simulink model "exampleModel"  (R2023b)
settings: Solver=VariableStepAuto  StartTime=0.0  StopTime=1  RelTol=1e-3
libraries: spsThreePhaseVIMeasurementLib x20, spsDistributedParametersLineLib x14, spsThreePhaseSeriesRLCLoadLib x14, spsLoadFlowBusLib x13, spsThreePhaseTransformerTwoWindingsLib x6, spsPower3phPhasorLib x1, spsThreePhaseSourceLib x1, sps_lib x1
settings Model: Creator=shivp  LastModifiedBy=shivp

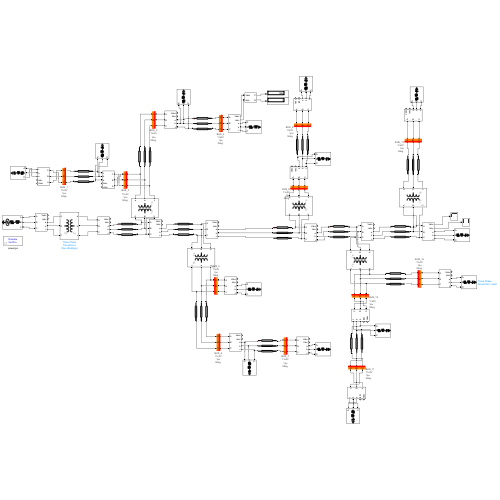
[thumbnail: Simulink's stored preview of the top-level diagram]
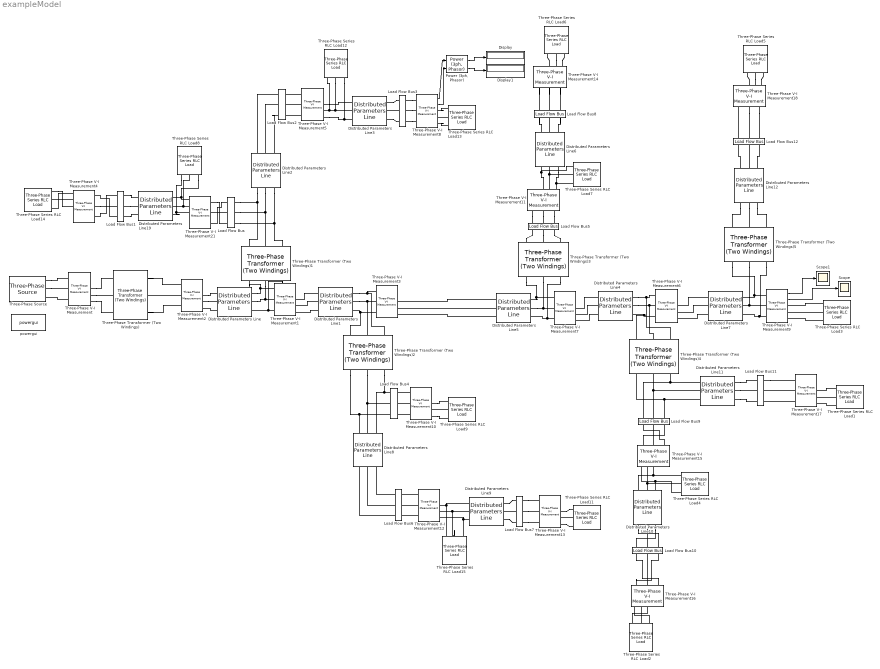
== system exampleModel ==
  Display : Display
  Display1 : Display
  Distributed Parameters Line : spsDistributedParametersLineLib/Distributed Parameters Line  Phases=3  Length=100  Frequency=60  Resistance=[0.01273 0.3864]  Inductance="[0.9337e-3  4.1264e-3]"  Capacitance=[12.74e-9 7.751e-9]  x1=[-0.0006 4.94077504274188 10377.8496125655 -30695.4420255601;-0.00055 5.1486824749925 10859.2496308345 -30528.5274235354;-0.0005 5.3553195468838 11337.9702917476 -30354.0803641771;-0.00045 5.56063527381028 11813.8934781449 -30172.1438896868;-0.0004 5.76457899718851 12286.9017631015 -29982.7628901672;-0.00035 5.96710039695644 12756.878438901 -29785.9840925461;-0.0003 6.16814950398906 13223.7075458309 -29581.8560490475;-0.00025 6.36767671242757 13687.2739007944 -29370.4291252116;-0.0002 6.56563279191888 14147.4631257301 -29151.7554874682;-0.00015 6.76196889976246 14604.1616758324 -28925.8890902654;-0.0001 6.95663659296153 15057.2568675681 -28692.8856627569;-5e-05 7.14958784017568 15506.6369064782 -28452.8026950519]  x2=[-0.0006 200.786537034863 2934.94544321627 -24233.8845899746;-0.00055 216.447490119636 3324.19339842984 -24183.5340234767;-0.0005 232.055038024995 3712.62115866332 -24127.2165318245;-0.00045 247.605329822035 4100.13288517904 -24064.9460105164;-0.0004 263.09452870894 4486.63296525695 -23996.7378238717;-0.00035 278.518812957654 4872.02603578562 -23922.6088012398;-0.0003 293.874376856837 5256.21700679164 -23842.5772328479;-0.00025 309.157431650868 5639.11108490171 -23756.6628652879;-0.0002 324.36420647466 6020.6137967314 -23664.8868966446;-0.00015 339.490949284071 6400.63101219513 -23567.2719712647;-0.0001 354.533927781658 6779.06896773129 -23463.8421741706;-5e-05 369.48943033757 7155.83428943706 -23354.6230251171]  x3=[-0.0006 -6.43137016476401 222.640411310815 145.145208722731;-0.00055 -6.37715378805683 220.308644649267 148.913129004531;-0.0005 -6.32136394407585 217.922520126202 152.644307199984;-0.00045 -6.26401439813027 215.482626482139 156.337822696701;-0.0004 -6.2051193003624 212.989565724328 159.992764175001;-0.00035 -6.14469318225637 210.443952978206 163.608229832763;-0.0003 -6.08275095305263 207.846416335627 167.183327607937;-0.00025 -6.01930789606939 205.19759669989 170.717175398642;-0.0002 -5.95437966493162 202.498147627605 174.208901280813;-0.00015 -5.88798227970884 199.748735167437 177.657643723337;-0.0001 -5.8201321229623 196.950037695771 181.06255180062;-5e-05 -5.75084593570292 194.102745749331 184.422785402543]  x4=[-0.0006 6.58204531239141 -184.73619828775 -350.009915302539;-0.00055 6.54912957666029 -179.156548049083 -353.150209345104;-0.0005 6.51459794120286 -173.532693612961 -356.203368857813;-0.00045 6.47845892618346 -167.866022581315 -359.168640519242;-0.0004 6.44072144836329 -162.157933120431 -362.045292692978;-0.00035 6.40139481890031 -156.409833615971 -364.832615608143;-0.0003 6.3604887410519 -150.623142325477 -367.529921534514;-0.00025 6.31801330778067 -144.799287028436 -370.136544952214;-0.0002 6.2739789992642 -138.939704673999 -372.651842715919;-0.00015 6.22839668030924 -133.045841026433 -375.075194213544;-0.0001 6.1812775976709 -127.119150308402 -377.406001519367;-5e-05 6.13263337727778 -121.161094842157 -379.643689541562]  x5=0.000565541566995742  V1=[14.16 3.243e+04 3.24e+04;314.2 314.2 314.2;0.3671 0.4058 -1.164]  V2=[1019 2.498e+04 2.442e+04;314.2 314.2 314.2;0.2092 0.1979 -1.367]  I1=[7.275 266.6 281.4;314.2 314.2 314.2;-1.074 2.234 0.6222]  I2=[6.892 399.1 404.5;314.2 314.2 314.2;1.883 -0.4011 -2.016]  nHarmo=1  Measurements=None  Decoupling=off  VsMag0=0  VrMag0=0  VsAngle0=0  VrAngle0=0  IsMag0=0  IrMag0=0  IsAngle0=0  IrAngle0=0
      settings: LibrarySourceBlock=sps_lib/Power Grid Elements/Distributed Parameters Line
  Distributed Parameters Line1 : spsDistributedParametersLineLib/Distributed Parameters Line  Phases=3  Length=100  Frequency=60  Resistance=[0.01273 0.3864]  Inductance="[0.9337e-3  4.1264e-3]"  Capacitance=[12.74e-9 7.751e-9]  x1=[-0.0006 200.786537034863 2934.94544321627 -24233.8845899746;-0.00055 216.447490119636 3324.19339842984 -24183.5340234767;-0.0005 232.055038024995 3712.62115866332 -24127.2165318245;-0.00045 247.605329822035 4100.13288517904 -24064.9460105164;-0.0004 263.09452870894 4486.63296525695 -23996.7378238717;-0.00035 278.518812957654 4872.02603578562 -23922.6088012398;-0.0003 293.874376856837 5256.21700679164 -23842.5772328479;-0.00025 309.157431650868 5639.11108490171 -23756.6628652879;-0.0002 324.36420647466 6020.6137967314 -23664.8868966446;-0.00015 339.490949284071 6400.63101219513 -23567.2719712647;-0.0001 354.533927781658 6779.06896773129 -23463.8421741706;-5e-05 369.48943033757 7155.83428943706 -23354.6230251171]  x2=[-0.0006 -9.4511266483093 -2063.31583954316 -18449.4745269581;-0.00055 0.255298879042691 -1766.85331668026 -18477.1445161307;-0.0005 9.96166141521642 -1469.95484919947 -18500.2555463735;-0.00045 19.6655660604955 -1172.69369235505 -18518.8019153854;-0.0004 29.3646185216113 -875.143190889432 -18532.7790471275;-0.00035 39.0564257024991 -577.376760936508 -18542.1834929517;-0.0003 48.7385962947587 -279.467871907298 -18547.0129324516;-0.00025 58.4087413676738 18.5099716375379 -18547.2661740353;-0.0002 68.0644749576452 316.483248123843 -18542.9431552193;-0.00015 77.7034146568914 614.378437104314 -18534.0449426437;-0.0001 87.3231822012721 912.122037398571 -18520.5737318095;-5e-05 96.9214040570896 1209.64058522847 -18502.5328465362]  x3=[-0.0006 2.35637752335621 200.746585968119 86.1206764107603;-0.00055 2.34192006818089 199.357183928959 89.1848960264509;-0.0005 2.32688477927164 197.918593487711 92.2271106035492;-0.00045 2.31127536636103 196.431169595039 95.2465695211299;-0.0004 2.29509568083813 194.895279250532 98.2425277728863;-0.00035 2.27834971479823 193.311301412151 101.214246150949;-0.0003 2.26104160005789 191.679626902725 104.160991428276;-0.00025 2.24317560713542 190.000658313525 107.082036539562;-0.0002 2.22475614419726 188.274809904927 109.976660760634;-0.00015 2.20578775597025 186.502507504201 112.84414988628;-0.0001 2.18627512262036 184.684188400446 115.683796406465;-5e-05 2.16622305859791 182.820301236692 118.494899680901]  x4=[-0.0006 -2.29653629180572 -206.26394733368 -243.453316618494;-0.00055 -2.2482852490429 -202.346734894282 -246.568009410702;-0.0005 -2.19947947553669 -198.379596425829 -249.621865236064;-0.00045 -2.15013101338141 -194.363510760375 -252.61413060135;-0.0004 -2.10025203857168 -190.299468806964 -255.544067209858;-0.00035 -2.04985485799818 -186.188473307137 -258.410952143569;-0.0003 -1.9989519064111 -182.03153858752 -261.214078041525;-0.00025 -1.94755574335208 -177.829690309553 -263.952753274354;-0.0002 -1.89567905005529 -173.583965216424 -266.626302114923;-0.00015 -1.84333462631855 -169.295410877271 -269.23406490506;-0.0001 -1.79053538734517 -164.965085428706 -271.775398218317;-5e-05 -1.73729436055733 -160.594057313737 -274.249675018726]  x5=0.000565541566995742  V1=[1019 2.498e+04 2.442e+04;314.2 314.2 314.2;0.2092 0.1979 -1.367]  V2=[618 1.897e+04 1.855e+04;314.2 314.2 314.2;-0.004469 -0.02884 -1.594]  I1=[2.523 218.7 213.9;314.2 314.2 314.2;1.947 2.059 0.4946]  I2=[3.821 322.4 315.2;314.2 314.2 314.2;-0.634 -0.6141 -2.179]  nHarmo=1  Measurements=None  Decoupling=off  VsMag0=0  VrMag0=0  VsAngle0=0  VrAngle0=0  IsMag0=0  IrMag0=0  IsAngle0=0  IrAngle0=0
      settings: LibrarySourceBlock=sps_lib/Power Grid Elements/Distributed Parameters Line
  Distributed Parameters Line10 : spsDistributedParametersLineLib/Distributed Parameters Line  Phases=3  Length=100  Frequency=60  Resistance=[0.01273 0.3864]  Inductance="[0.9337e-3  4.1264e-3]"  Capacitance=[12.74e-9 7.751e-9]  x1=[-0.0006 -31.2534203294304 -3259.14632862606 -2098.05285456964;-0.00055 -31.121311210234 -3225.34530243776 -2147.64844888902;-0.0005 -30.9815233731746 -3190.74847055797 -2196.71414308959;-0.00045 -30.8340913088094 -3155.36436923726 -2245.23783094549;-0.0004 -30.6790513937942 -3119.20172897317 -2293.20753996283;-0.00035 -30.5164418819081 -3082.26947235608 -2340.61143433367;-0.0003 -30.3463028946149 -3044.57671186767 -2387.43781785642;-0.00025 -30.1686764111639 -3006.13274763258 -2433.67513682161;-0.0002 -29.9836062582321 -2966.94706512375 -2479.31198286265;-0.00015 -29.7911380991104 -2927.02933282198 -2524.33709577066;-0.0001 -29.5913194224371 -2886.38939983042 -2568.73936627276;-5e-05 -29.3841995304807 -2845.03729344442 -2612.5078387731]  x2=[-0.0006 -31.9626959429525 -2654.70923607677 -3040.23236273384;-0.00055 -31.1478015841112 -2605.78900431863 -3080.34012920064;-0.0005 -30.3252219713036 -2556.22583311494 -3119.68786783269;-0.00045 -29.4951600637406 -2506.03195143655 -3158.26587016424;-0.0004 -28.6578206667774 -2455.2197438727 -3196.06461765047;-0.00035 -27.8134103813809 -2403.8017475753 -3233.07478401604;-0.0003 -26.9621375531538 -2351.79064916554 -3269.28723755619;-0.00025 -26.1042122209286 -2299.19928160369 -3304.69304338987;-0.0002 -25.2398460649435 -2246.04062102277 -3339.28346566427;-0.00015 -24.3692523546139 -2192.32778352684 -3373.0499697103;-0.0001 -23.4926458959107 -2138.07402195483 -3405.98422414832;-5e-05 -22.6102429783607 -2083.29272261059 -3438.07810294388]  x3=[-0.0006 -0.345240872027474 -44.4331799500981 -28.7697264815166;-0.00055 -0.343762803006474 -43.96968801251 -29.4458458734078;-0.0005 -0.342199915657665 -43.4953472123374 -30.1146999434374;-0.00045 -0.340552595600116 -43.010274586075 -30.7761236618718;-0.0004 -0.338821249285399 -42.5145898181351 -31.4299538323058;-0.00035 -0.337006303897313 -42.008415211317 -32.076029131928;-0.0003 -0.335108207246473 -41.4918756566308 -32.714190151326;-0.00025 -0.333127427659828 -40.9650986024827 -33.344279433817;-0.0002 -0.331064453865099 -40.4282140232284 -33.9661415142989;-0.00015 -0.328919794870204 -39.8813543871042 -34.5796229576084;-0.0001 -0.326693979837657 -39.3246546235424 -35.1845723963791;-5e-05 -0.324387557954011 -38.7582520898798 -35.7808405683891]  x4=[-0.0006 0.254867368595789 21.6219762320696 11.0058318246452;-0.00055 0.254519474301124 21.4445338180896 11.3354955184404;-0.0005 0.254108781134632 21.2618002862713 11.662362348333;-0.00045 0.253635390428706 21.0738207233796 11.9863516648239;-0.0004 0.25309941898542 20.8806415105588 12.307383528397;-0.00035 0.252500999047707 20.6823103118889 12.6253787292439;-0.0003 0.251840278266732 20.4788760626257 12.940258806807;-0.00025 0.251117419665462 20.270388957126 13.2519460691387;-0.0002 0.250332601598441 20.0569004364634 13.5603636120709;-0.00015 0.249486017707782 19.8384631757361 13.86543533819;-0.0001 0.248577876875393 19.6151310710694 14.1670859756123;-5e-05 0.247608403171435 19.3869592263184 14.4652410965568]  x5=0.000565541566995742  V1=[32.3 3891 3805;314.2 314.2 314.2;-1.304 -0.9126 -2.477]  V2=[60.72 4077 3986;314.2 314.2 314.2;-0.5435 -0.629 -2.194]  I1=[0.3571 53.15 51.96;314.2 314.2 314.2;-1.301 -0.9099 -2.475]  I2=[0.2557 24.32 23.78;314.2 314.2 314.2;1.661 2.126 0.5614]  nHarmo=1  Measurements=None  Decoupling=off  VsMag0=0  VrMag0=0  VsAngle0=0  VrAngle0=0  IsMag0=0  IrMag0=0  IsAngle0=0  IrAngle0=0
      settings: LibrarySourceBlock=sps_lib/Power Grid Elements/Distributed Parameters Line
  Distributed Parameters Line11 : spsDistributedParametersLineLib/Distributed Parameters Line  Phases=3  Length=100  Frequency=60  Resistance=[0.01273 0.3864]  Inductance="[0.9337e-3  4.1264e-3]"  Capacitance=[12.74e-9 7.751e-9]  x1=[-0.0006 -31.253420329437 187.39390622673 3871.52994252577;-0.00055 -31.1213112102406 247.245463917248 3867.05519233241;-0.0005 -30.9815233731812 307.036017489159 3861.62630413434;-0.00045 -30.834091308816 366.750814518032 3855.24461742848;-0.0004 -30.6790513938007 426.375121271234 3847.91170680052;-0.00035 -30.5164418819145 485.89422634325 3839.62938153646;-0.0003 -30.3463028946213 545.293444285507 3830.39968517611;-0.00025 -30.1686764111703 604.558119229787 3820.22489500894;-0.0002 -29.9836062582384 663.673628504345 3809.10752151218;-0.00015 -29.7911380991167 722.625386241831 3797.05030773138;-0.0001 -29.5913194224434 781.398846978137 3784.05622860364;-5e-05 -29.384199530487 839.979509241274 3770.12849022354]  x2=[-0.0006 -31.9626959429525 1305.5638414967 3819.16181947058;-0.00055 -31.1478015841112 1364.75830202508 3796.84953924242;-0.0005 -30.3252219713036 1423.61602886375 3773.60044320392;-0.00045 -29.4951600637406 1482.12249974932 3749.42026772166;-0.0004 -28.6578206667774 1540.26327908556 3724.31497889212;-0.00035 -27.8134103813809 1598.02402150513 3698.29077106966;-0.0003 -26.9621375531538 1655.39047540914 3671.35406533815;-0.00025 -26.1042122209286 1712.34848648349 3643.51150792666;-0.0002 -25.2398460649435 1768.88400119122 3614.76996856963;-0.00015 -24.3692523546139 1824.98307024003 3585.13653881182;-0.0001 -23.4926458959107 1880.63185202407 3554.61853025861;-5e-05 -22.6102429783607 1935.81661603912 3523.22347277195]  x3=[-0.0006 -0.345240872027459 2.69872401787422 52.8651258484685;-0.00055 -0.343762803006458 3.51600655603732 52.8017897520135;-0.0005 -0.342199915657649 4.33242157219386 52.7254256040274;-0.00045 -0.340552595600099 5.14776762815486 52.636052246221;-0.0004 -0.338821249285382 5.96184354948133 52.5336917301329;-0.00035 -0.337006303897295 6.77444847512094 52.418369311689;-0.0003 -0.335108207246455 7.58538190696757 52.2901134449703;-0.00025 -0.333127427659809 8.39444375933115 52.1489557751928;-0.0002 -0.33106445386508 9.20143440830588 51.9949311308993;-0.00015 -0.328919794870184 10.0061547410244 51.8280775153662;-0.0001 -0.326693979837637 10.8084062047858 51.6484360972263;-5e-05 -0.324387557953991 11.6079908560459 51.4560512003116]  x4=[-0.0006 0.254867368595761 1.27965816611283 -24.228096609318;-0.00055 0.254519474301095 0.905439825590797 -24.2392588180001;-0.0005 0.254108781134602 0.530998081340184 -24.2444403522685;-0.00045 0.253635390428675 0.156425321258497 -24.2436399336574;-0.0004 0.253099418985388 -0.21818603443057 -24.2368577596581;-0.00035 0.252500999047674 -0.592743555980428 -24.2240955036704;-0.0003 0.251840278266699 -0.967154826927261 -24.2053563145901;-0.00025 0.251117419665428 -1.3413274668924 -24.1806448160318;-0.0002 0.250332601598405 -1.71516915437579 -24.1499671051878;-0.00015 0.249486017707745 -2.08858764953497 -24.1133307513243;-0.0001 0.248577876875355 -2.46149081694384 -24.0707447939135;-5e-05 0.247608403171397 -2.8337866483257 -24.022219740403]  x5=0.000565541566995742  V1=[32.3 3817 3880;314.2 314.2 314.2;-1.304 0.1293 1.717]  V2=[60.72 3998 4064;314.2 314.2 314.2;-0.5435 0.4128 2]  I1=[0.3571 52.12 52.99;314.2 314.2 314.2;-1.301 0.1319 1.719]  I2=[0.2557 23.85 24.24;314.2 314.2 314.2;1.661 -3.115 -1.528]  nHarmo=1  Measurements=None  Decoupling=off  VsMag0=0  VrMag0=0  VsAngle0=0  VrAngle0=0  IsMag0=0  IrMag0=0  IsAngle0=0  IrAngle0=0
      settings: LibrarySourceBlock=sps_lib/Power Grid Elements/Distributed Parameters Line
  Distributed Parameters Line12 : spsDistributedParametersLineLib/Distributed Parameters Line  Phases=3  Length=100  Frequency=60  Resistance=[0.01273 0.3864]  Inductance="[0.9337e-3  4.1264e-3]"  Capacitance=[12.74e-9 7.751e-9]  x1=[-0.0006 -13.9948706374657 -919.303427512541 3469.68312771773;-0.00055 -14.107672519494 -865.812114028127 3483.03655716339;-0.0005 -14.2169935444258 -812.107174360002 3495.53059945637;-0.00045 -14.3228067389339 -758.201859398424 3507.16217187868;-0.0004 -14.4250859951959 -704.109469473257 3517.92840451387;-0.00035 -14.5238060773359 -649.843351072314 3527.82664095514;-0.0003 -14.6189426276506 -595.416893548309 3536.85443896076;-0.00025 -14.7104721726198 -540.843525815234 3545.00957105666;-0.0002 -14.798372128698 -486.136713034981 3552.29002508601;-0.00015 -14.8826208078863 -431.309953295005 3558.69400470573;-0.0001 -14.9631974230836 -376.376774277884 3564.21992982967;-5e-05 -15.0400820932159 -321.350729923556 3568.86643701849]  x2=[-0.0006 -28.5037047462179 71.306703847752 3746.70935246665;-0.00055 -28.3711521317178 129.213636434848 3744.1363373644;-0.0005 -28.2315993599558 187.088687490618 3740.63951264562;-0.00045 -28.0850808634902 244.917577212219 3736.21974109948;-0.0004 -27.9316327935677 302.686037186423 3730.87811323849;-0.00035 -27.7712930112033 360.379813910139 3724.61594702938;-0.0003 -27.6041010778393 417.984672307252 3717.43478756796;-0.00025 -27.4300982455832 475.486399240912 3709.33640669789;-0.0002 -27.2493274470305 532.870807020415 3700.32280257345;-0.00015 -27.0618332846706 590.123736901803 3690.3961991666;-0.0001 -26.8676620198827 647.231062581322 3679.55904571818;-5e-05 -26.6668615615208 704.178693680874 3667.81401613366]  x3=[-0.0006 -0.154985241892026 -12.4308431243015 47.4184090726545;-0.00055 -0.156224478566297 -11.6997862553303 47.5987825840961;-0.0005 -0.157425169188118 -10.9658426391682 47.767411808171;-0.00045 -0.158587017505046 -10.2291933654204 47.9242551381413;-0.0004 -0.159709736848393 -9.49002019127238 48.0692738752623;-0.00035 -0.160793050203961 -8.74850549664436 48.2024322383305;-0.0003 -0.161836690280388 -8.00483223919175 48.3236973725125;-0.00025 -0.162840399575104 -7.25918390916299 48.4330393574507;-0.0002 -0.163803930437857 -6.51174448412615 48.5304312146467;-0.00015 -0.164727045131826 -5.76269838357518 48.6158489141168;-0.0001 -0.165609515892272 -5.01223042342716 48.689271380322;-5e-05 -0.166451124982741 -4.26052577042177 48.7506804973673]  x4=[-0.0006 0.098898525106131 7.89349892269427 -21.004432828506;-0.00055 0.100084430701719 7.56999516148253 -21.1224544565239;-0.0005 0.101245641961626 7.24462361723696 -21.2352644349667;-0.00045 0.102381872374351 6.91746457051747 -21.3428349296603;-0.0004 0.10349284159204 6.58859874292344 -21.4451393991946;-0.00035 0.104578275499663 6.25810727717692 -21.5421526014727;-0.0003 0.105637906282645 5.92607171710183 -21.6338505999386;-0.00025 0.106671472492945 5.59257398750425 -21.7202107694831;-0.0002 0.107678719113567 5.25769637395874 -21.8012118020268;-0.00015 0.10865939762148 4.92152150250556 -21.8768337117769;-0.0001 0.109613266048934 4.58413231926394 -21.9470578401587;-5e-05 0.11054008904317 4.24561206996638 -22.0118668604193]  x5=0.000565541566995742  V1=[15.78 3520 3579;314.2 314.2 314.2;-2.04 -0.1841 1.403]  V2=[29.66 3688 3749;314.2 314.2 314.2;-1.279 0.09948 1.687]  I1=[0.1745 48.08 48.88;314.2 314.2 314.2;-2.037 -0.1814 1.406]  I2=[0.1249 22 22.36;314.2 314.2 314.2;0.9246 2.855 -1.841]  nHarmo=1  Measurements=None  Decoupling=off  VsMag0=0  VrMag0=0  VsAngle0=0  VrAngle0=0  IsMag0=0  IrMag0=0  IsAngle0=0  IrAngle0=0
      settings: LibrarySourceBlock=sps_lib/Power Grid Elements/Distributed Parameters Line
  Distributed Parameters Line19 : spsDistributedParametersLineLib/Distributed Parameters Line  Phases=3  Length=100  Frequency=60  Resistance=[0.01273 0.3864]  Inductance="[0.9337e-3  4.1264e-3]"  Capacitance=[12.74e-9 7.751e-9]  x1=[-0.0006 -96.5409517097259 5973.89106489545 4979.15177398064;-0.00055 -94.1120389876083 6051.66956004539 4881.77212845539;-0.0005 -91.6599055280992 6127.95489628446 4783.18797870496;-0.00045 -89.1851563584376 6202.72825134744 4683.42364889317;-0.0004 -86.6884020859507 6275.97117602781 4582.50375437559;-0.00035 -84.1702587473955 6347.66559872986 4480.45319562609;-0.0003 -81.631347656961 6417.79382992759 4377.29715209302;-0.00025 -79.0722952529682 6486.3385665293 4273.06107598659;-0.0002 -76.4937329433059 6553.28289614688 4167.77068599884;-0.00015 -73.8962969496402 6618.61030126871 4061.45196095801;-0.0001 -71.2806281504361 6682.3046633351 3954.13113341862;-5e-05 -68.6473719228309 6744.35026671528 3845.834683189]  x2=[-0.0006 68.0412810259189 7473.03807820244 3202.33927910117;-0.00055 73.2889661597856 7523.58354001883 3081.70422208403;-0.0005 78.5185683378987 7572.27267017452 2960.30880066263;-0.00045 83.728797234173 7619.0934553552 2838.18296734071;-0.0004 88.9183673025907 7664.0343432327 2715.35685484025;-0.00035 94.0859980943905 7707.08424531542 2591.86076866661;-0.0003 99.2304145739996 7748.23253968419 2467.72517963114;-0.00025 104.350347433629 7787.46907361308 2342.98071633297;-0.0002 109.444533406457 7824.78416607446 2217.65815760182;-0.00015 114.511715578321 7860.16861012761 2091.78842490381;-0.0001 119.550643697841 7893.61367519045 1965.40257471205;-5e-05 124.560074484904 7925.11110919361 1838.53179084394]  x3=[-0.0006 -1.06184548840488 81.7697475785311 67.7761452130824;-0.00055 -1.0349383777841 82.8285325706211 66.44337440146;-0.0005 -1.00777591160473 83.8668808616892 65.0942096814175;-0.00045 -0.980364791798835 84.8845362548318 63.7289839391618;-0.0004 -0.952711781650081 85.8812476588081 62.3480340237163;-0.00035 -0.924823704124937 86.8567691499932 60.9517006638091;-0.0003 -0.896707440189235 87.8108600330563 59.540328383803;-0.00025 -0.868369927110387 88.7432849003484 58.1142654186893;-0.0002 -0.839818156745723 89.6538136899856 56.6738636281659;-0.00015 -0.81105917381735 90.5422217426136 55.2194784098215;-0.0001 -0.782100074173978 91.408289856839 53.7514686114462;-5e-05 -0.752948003040117 92.2518043433138 52.2701964424916]  x4=[-0.0006 0.96623222764616 -33.9273887860384 -34.9003273923412;-0.00055 0.949390278302067 -34.4714181256832 -34.3446948123242;-0.0005 0.932314081112835 -35.0069421587123 -33.7805881927728;-0.00045 0.915007849374603 -35.5338287525838 -33.2081467185547;-0.0004 0.897475853141095 -36.0519479059148 -32.627511631038;-0.00035 0.879722418170043 -36.5611717805569 -32.0388261932422;-0.0003 0.861751924855877 -37.0613747331386 -31.4422356544905;-0.00025 0.843568807148924 -37.5524333460662 -30.8378872145714;-0.0002 0.825177551461397 -38.0342264579748 -30.2259299874192;-0.00015 0.806582695560445 -38.5066351936232 -29.606514964323;-0.0001 0.787788827448518 -38.9695429932248 -28.979794976671;-5e-05 0.768800584231356 -39.4228356412065 -28.3459246582426]  x5=0.000565541566995742  V1=[181.7 7789 7921;314.2 314.2 314.2;-0.5495 0.9542 2.542]  V2=[341.5 8160 8298;314.2 314.2 314.2;0.2114 1.238 2.826]  I1=[2.008 106.4 108.2;314.2 314.2 314.2;-0.5463 0.9569 2.545]  I2=[1.438 48.67 49.5;314.2 314.2 314.2;2.415 -2.29 -0.7024]  nHarmo=1  Measurements=None  Decoupling=off  VsMag0=0  VrMag0=0  VsAngle0=0  VrAngle0=0  IsMag0=0  IrMag0=0  IsAngle0=0  IrAngle0=0
      settings: LibrarySourceBlock=sps_lib/Power Grid Elements/Distributed Parameters Line
  Distributed Parameters Line2 : spsDistributedParametersLineLib/Distributed Parameters Line  Phases=3  Length=100  Frequency=60  Resistance=[0.01273 0.3864]  Inductance="[0.9337e-3  4.1264e-3]"  Capacitance=[12.74e-9 7.751e-9]  x1=[-0.0006 68.0412810259189 963.211871862868 -8073.01045872234;-0.00055 73.2889661597856 1092.95762673489 -8056.46658419278;-0.0005 78.5185683378987 1222.43371066678 -8037.93489708508;-0.00045 83.728797234173 1351.60817737224 -8017.41996981571;-0.0004 88.9183673025907 1480.44915498448 -7994.92686413603;-0.00035 94.0859980943905 1608.92485392017 -7970.46112988328;-0.0003 99.2304145739996 1737.00357472301 -7944.0288036113;-0.00025 104.350347433629 1864.65371588512 -7915.63640710108;-0.0002 109.444533406457 1991.84378164426 -7885.29094575162;-0.00015 114.511715578321 2118.54238975487 -7852.99990685144;-0.0001 119.550643697841 2244.71827923124 -7818.7712577312;-5e-05 124.560074484904 2370.34031806066 -7782.61344379791]  x2=[-0.0006 2087.33596012298 -628.82209039192 -6402.97812602283;-0.00055 2162.21893486438 -491.528832065564 -6413.85133834206;-0.0005 2236.56841443757 -354.114296354799 -6423.14202881608;-0.00045 2310.366054221 -216.612388240135 -6430.84790510602;-0.0004 2383.59364575129 -79.0570342599129 -6436.96706590223;-0.00035 2456.23312121598 58.5178258605571 -6441.49800139332;-0.0003 2528.2665579114 196.078247583117 -6444.43959363878;-0.00025 2599.67618266493 333.590289932067 -6445.79111684472;-0.0002 2670.44437622018 471.020023868596 -6445.55223754303;-0.00015 2740.55367758431 608.333540662258 -6443.72301467359;-0.0001 2809.98678833628 745.496960257453 -6440.30389956978;-5e-05 2878.72657689496 882.476439632814 -6435.29573584708]  x3=[-0.0006 -26.6808406064646 -16.3698197682876 31.4708857070339;-0.00055 -26.3068314629707 -16.7265120702519 32.3510666584731;-0.0005 -25.9263315024508 -17.079077355647 33.2232654682938;-0.00045 -25.5394346075767 -17.4274286342643 34.0872669344905;-0.0004 -25.1462362393679 -17.7714799556384 34.9428578776299;-0.00035 -24.7468334136383 -18.1111464302537 35.7898271934492;-0.0003 -24.3413246770587 -18.4463442504903 36.6279659049431;-0.00025 -23.9298100828421 -18.7769907113017 37.4570672139261;-0.0002 -23.512391166057 -19.1030042306211 38.2769265520561;-0.00015 -23.0891709185751 -19.4243043694911 39.0873416313094;-0.0001 -22.6602537636597 -19.74081185191 39.8881124938916;-5e-05 -22.2257455302008 -20.0524485843925 40.6790415615746]  x4=[-0.0006 28.9112968002983 14.2025818885613 -84.804264208584;-0.00055 28.6469314818365 15.5436737884218 -85.7090067587712;-0.0005 28.3754979616847 16.8809305193601 -86.592601894032;-0.00045 28.0970632120027 18.2140221332874 -87.4548316004884;-0.0004 27.8116959323984 19.5426197097956 -88.2954831358622;-0.00035 27.5194665329782 20.866395437313 -89.1143490819658;-0.0003 27.2204471169735 22.1850226939867 -89.9112273958801;-0.00025 26.9147114629511 23.4981761282724 -90.685921459805;-0.0002 26.6023350066086 24.8055317392091 -91.4382401295723;-0.00015 26.2833948221626 26.1067669563623 -92.1679977818074;-0.0001 25.957969603331 27.401560719413 -92.8750143597291;-5e-05 25.6261396439173 28.6895935573745 -93.5591154175763]  x5=0.000565541566995742  V1=[341.5 8324 8133;314.2 314.2 314.2;0.2114 0.1961 -1.369]  V2=[5219 8758 6446;314.2 314.2 314.2;0.4223 0.008285 -1.606]  I1=[35.62 28.1 64.48;314.2 314.2 314.2;-0.8357 -2.44 0.59]  I2=[33.34 86.66 102.9;314.2 314.2 314.2;2.103 0.2448 -2.093]  nHarmo=1  Measurements=None  Decoupling=off  VsMag0=0  VrMag0=0  VsAngle0=0  VrAngle0=0  IsMag0=0  IrMag0=0  IsAngle0=0  IrAngle0=0
      settings: LibrarySourceBlock=sps_lib/Power Grid Elements/Distributed Parameters Line
  Distributed Parameters Line3 : spsDistributedParametersLineLib/Distributed Parameters Line  Phases=3  Length=100  Frequency=60  Resistance=[0.01273 0.3864]  Inductance="[0.9337e-3  4.1264e-3]"  Capacitance=[12.74e-9 7.751e-9]  x1=[-0.0006 2087.33596012298 -628.82209039192 -6402.97812602283;-0.00055 2162.21893486438 -491.528832065564 -6413.85133834206;-0.0005 2236.56841443757 -354.114296354799 -6423.14202881608;-0.00045 2310.366054221 -216.612388240135 -6430.84790510602;-0.0004 2383.59364575129 -79.0570342599129 -6436.96706590223;-0.00035 2456.23312121598 58.5178258605571 -6441.49800139332;-0.0003 2528.2665579114 196.078247583117 -6444.43959363878;-0.00025 2599.67618266493 333.590289932067 -6445.79111684472;-0.0002 2670.44437622018 471.020023868596 -6445.55223754303;-0.00015 2740.55367758431 608.333540662258 -6443.72301467359;-0.0001 2809.98678833628 745.496960257453 -6440.30389956978;-5e-05 2878.72657689496 882.476439632814 -6435.29573584708]  x2=[-0.0006 2032.53535980036 -653.518029025961 -6422.47366898926;-0.00055 2107.95992574584 -515.788326387144 -6433.64359200742;-0.0005 2182.86438412173 -377.931360696697 -6443.22610973794;-0.00045 2257.23025337374 -239.981146098108 -6451.21885783794;-0.0004 2331.03918483639 -101.971719742633 -6457.61986421643;-0.00035 2404.27296726027 36.0628666088533 -6462.42754952086;-0.0003 2476.91353130539 174.088554987623 -6465.64072752682;-0.00025 2548.94295399951 312.071289620394 -6467.25860543073;-0.0002 2620.34346316038 449.977025332073 -6467.28078404542;-0.00015 2691.09744178076 587.771735945902 -6465.70725789864;-0.0001 2761.18743237513 725.421422678904 -6462.53841523443;-5e-05 2830.5961412871 862.892122530573 -6457.7750379173]  x3=[-0.0006 1.83174607129767 -5.03528335408262 -22.8009929422156;-0.00055 1.92951356512839 -4.54412167364308 -22.8720657163869;-0.0005 2.02680498035884 -4.05183879917573 -22.9374951505846;-0.00045 2.12359631178813 -3.55855619411364 -22.9972651010751;-0.0004 2.21986367760354 -3.06439556855847 -23.0513608205174;-0.00035 2.31558332527303 -2.5694788492503 -23.0997689616021;-0.0003 2.41073163740582 -2.07392814948401 -23.1424775803447;-0.00025 2.50528513757964 -1.57786573897969 -23.1794761390328;-0.0002 2.59922049613315 -1.08141401371439 -23.2107555088255;-0.00015 2.69251453592221 -0.584695465722753 -23.2363079720064;-0.0001 2.78514423803848 -0.0878326528739325 -23.2561272238876;-5e-05 2.87708674748903 0.409051831367717 -23.2702083743651]  x4=[-0.0006 2.45325998706616 -3.18193840029037 -24.1069926895373;-0.00055 2.56130378368838 -2.66437550790577 -24.157353960326;-0.0005 2.66871561692759 -2.1461552207325 -24.2017547654993;-0.00045 2.77546898452117 -1.62740540187212 -24.2401841498228;-0.0004 2.88153754667306 -1.10825404508022 -24.2726326314211;-0.00035 2.98689513255267 -0.588829243185862 -24.2990922041167;-0.0003 3.0915157467522 -0.0692591564865859 -24.3195563394061;-0.00025 3.19537357570056 0.450328018873207 -24.3340199880701;-0.0002 3.29844299403252 0.969804082532746 -24.3424795814197;-0.00015 3.40069857091136 1.48904086154641 -24.344933032177;-0.0001 3.50211507630357 2.00791024200848 -24.3413797349897;-5e-05 3.60266748720398 2.52628420066335 -24.3318205665806]  x5=0.000565541566995742  V1=[5219 8758 6446;314.2 314.2 314.2;0.4223 0.008285 -1.606]  V2=[5229 8788 6467;314.2 314.2 314.2;0.41 0.005707 -1.609]  I1=[6.502 31.63 23.28;314.2 314.2 314.2;0.2964 -0.07971 -1.694]  I2=[7.321 33.08 24.34;314.2 314.2 314.2;0.3525 -0.0162 -1.631]  nHarmo=1  Measurements=None  Decoupling=off  VsMag0=0  VrMag0=0  VsAngle0=0  VrAngle0=0  IsMag0=0  IrMag0=0  IsAngle0=0  IrAngle0=0
      settings: LibrarySourceBlock=sps_lib/Power Grid Elements/Distributed Parameters Line
  Distributed Parameters Line4 : spsDistributedParametersLineLib/Distributed Parameters Line  Phases=3  Length=100  Frequency=60  Resistance=[0.01273 0.3864]  Inductance="[0.9337e-3  4.1264e-3]"  Capacitance=[12.74e-9 7.751e-9]  x1=[-0.0006 -85.8427686297971 -5484.91312356955 -13494.6318129038;-0.00055 -80.370432368254 -5267.95419020034 -13575.9280426568;-0.0005 -74.8782659051327 -5049.69546796078 -13653.8746153063;-0.00045 -69.3676243503268 -4830.19080892472 -13728.4522987018;-0.0004 -63.8398673721825 -4609.49437258225 -13799.6426919159;-0.00035 -58.2963588620205 -4387.6606124767 -13867.4282297842;-0.0003 -52.7384665976165 -4164.74426276899 -13931.7921872395;-0.00025 -47.1675619057221 -3940.80032473284 -13992.7186834386;-0.0002 -41.5850193237109 -3715.88405318404 -14050.19268568;-0.00015 -35.9922162604316 -3490.05094284707 -14104.2000131138;-0.0001 -30.3905326563531 -3263.35671466271 -14154.7273402401;-5e-05 -24.7813506430849 -3035.85730203966 -14201.7622001969]  x2=[-0.0006 -95.754041116279 -7950.01158904029 -9140.45194809051;-0.00055 -93.3058973660337 -7802.93392827206 -9260.55415698169;-0.0005 -90.8347317817795 -7653.93101031483 -9378.37146270328;-0.00045 -88.3411540866474 -7503.03959940903 -9493.87479559802;-0.0004 -85.8257795336214 -7350.29692575247 -9607.03565694686;-0.00035 -83.2892287537342 -7195.74067631434 -9717.8261260005;-0.0003 -80.7321276029355 -7039.40898553651 -9826.21886686851;-0.00025 -78.1551070076716 -6881.34042592443 -9932.18713526398;-0.0002 -75.5588028092135 -6721.57399852996 -10035.7047851023;-0.00015 -72.9438556067728 -6560.14912332842 -10136.7462749524;-0.0001 -70.3109105994435 -6397.10562949233 -10235.2866743386;-5e-05 -67.6606174270086 -6232.4837455641 -10331.3016698917]  x3=[-0.0006 1.1620076929778 125.414435966357 40.665892619007;-0.00055 1.16160345551954 124.757477557021 42.5830940659025;-0.0005 1.16091260979007 124.069737106883 44.4897887715218;-0.00045 1.15993532624525 123.35138430561 46.3855062874767;-0.0004 1.15867184601516 122.602596396006 48.2697788738364;-0.00035 1.15712248084465 121.823558130283 50.1421416145351;-0.0003 1.15528761301638 121.014461724477 52.0021325320835;-0.00025 1.15316769525654 120.175506811018 53.8492927015541;-0.0002 1.15076325062311 119.306900389479 55.683166363815;-0.00015 1.14807487237683 118.408856775496 57.5033010379806;-0.0001 1.14510322383481 117.481597547893 59.3092476330555;-5e-05 1.14184903820685 116.52535149401 61.1005605587403]  x4=[-0.0006 -1.46097545043501 -179.47695710863 -121.384323906679;-0.00055 -1.45047049704238 -177.521638196142 -124.114215626958;-0.0005 -1.43960766175845 -175.522518475743 -126.813484021692;-0.00045 -1.4283896248253 -173.480091200309 -129.481463086795;-0.0004 -1.41681915412568 -171.39486030821 -132.117494538354;-0.00035 -1.4048991045001 -169.267340298967 -134.720927975052;-0.0003 -1.39263241704243 -167.098056106306 -137.291121038645;-0.00025 -1.38002211837427 -164.887542968643 -139.827439572452;-0.0002 -1.36707131989811 -162.636346297017 -142.329257777828;-0.00015 -1.3537832170297 -160.345021540523 -144.795958368566;-0.0001 -1.34016108840958 -158.014134049258 -147.226932723205;-5e-05 -1.32620829509415 -155.644258934832 -149.621581035198]  x5=0.000565541566995742  V1=[358.2 1.482e+04 1.449e+04;314.2 314.2 314.2;-0.2312 -0.2989 -1.864]  V2=[182.3 1.224e+04 1.196e+04;314.2 314.2 314.2;-0.5422 -0.6271 -2.192]  I1=[1.162 131.9 129;314.2 314.2 314.2;1.596 1.966 0.401]  I2=[1.602 217.6 212.8;314.2 314.2 314.2;-1.137 -0.8896 -2.454]  nHarmo=1  Measurements=None  Decoupling=off  VsMag0=0  VrMag0=0  VsAngle0=0  VrAngle0=0  IsMag0=0  IrMag0=0  IsAngle0=0  IrAngle0=0
      settings: LibrarySourceBlock=sps_lib/Power Grid Elements/Distributed Parameters Line
  Distributed Parameters Line5 : spsDistributedParametersLineLib/Distributed Parameters Line  Phases=3  Length=100  Frequency=60  Resistance=[0.01273 0.3864]  Inductance="[0.9337e-3  4.1264e-3]"  Capacitance=[12.74e-9 7.751e-9]  x1=[-0.0006 -9.4511266483093 -2063.31583954316 -18449.4745269581;-0.00055 0.255298879042691 -1766.85331668026 -18477.1445161307;-0.0005 9.96166141521642 -1469.95484919947 -18500.2555463735;-0.00045 19.6655660604955 -1172.69369235505 -18518.8019153854;-0.0004 29.3646185216113 -875.143190889432 -18532.7790471275;-0.00035 39.0564257024991 -577.376760936508 -18542.1834929517;-0.0003 48.7385962947587 -279.467871907298 -18547.0129324516;-0.00025 58.4087413676738 18.5099716375379 -18547.2661740353;-0.0002 68.0644749576452 316.483248123843 -18542.9431552193;-0.00015 77.7034146568914 614.378437104314 -18534.0449426437;-0.0001 87.3231822012721 912.122037398571 -18520.5737318095;-5e-05 96.9214040570896 1209.64058522847 -18502.5328465362]  x2=[-0.0006 -85.8427686297971 -5484.91312356955 -13494.6318129038;-0.00055 -80.370432368254 -5267.95419020034 -13575.9280426568;-0.0005 -74.8782659051327 -5049.69546796078 -13653.8746153063;-0.00045 -69.3676243503268 -4830.19080892472 -13728.4522987018;-0.0004 -63.8398673721825 -4609.49437258225 -13799.6426919159;-0.00035 -58.2963588620205 -4387.6606124767 -13867.4282297842;-0.0003 -52.7384665976165 -4164.74426276899 -13931.7921872395;-0.00025 -47.1675619057221 -3940.80032473284 -13992.7186834386;-0.0002 -41.5850193237109 -3715.88405318404 -14050.19268568;-0.00015 -35.9922162604316 -3490.05094284707 -14104.2000131138;-0.0001 -30.3905326563531 -3263.35671466271 -14154.7273402401;-5e-05 -24.7813506430849 -3035.85730203966 -14201.7622001969]  x3=[-0.0006 1.63217458490605 156.675952932982 54.5703921027448;-0.00055 1.62769522557648 155.794703782385 56.9646656326633;-0.0005 1.62281425680573 154.875014619837 59.3448839837175;-0.00045 1.6175328828998 153.917112364875 61.7104598726452;-0.0004 1.61185240695868 152.921233365549 64.0608096289928;-0.00035 1.60577423055481 151.887623340099 66.3953533391269;-0.0003 1.59929985338726 150.816537316333 68.7135149893196;-0.00025 1.59243087291173 149.708239568701 71.0147226078711;-0.0002 1.58516898394636 148.563003553088 73.2984084062352;-0.00015 1.5775159782536 147.381111839344 75.5640089191127;-0.0001 1.56947374409808 146.162856041564 77.8109651434779;-5e-05 1.56104426578074 144.908536746138 80.0387226765044]  x4=[-0.0006 -1.87248471190371 -190.980297717364 -170.715353830612;-0.00055 -1.84817646152045 -188.232110567907 -173.611166455173;-0.0005 -1.82341220125017 -185.437479961745 -176.464143122212;-0.00045 -1.79819804130352 -182.597095432162 -179.273579902424;-0.0004 -1.77254020289721 -179.711657801541 -182.038783609324;-0.00035 -1.74644501671891 -176.781879008441 -184.759071970273;-0.0003 -1.71991892136536 -173.808481931939 -187.433773794823;-0.00025 -1.69296846175366 -170.792200213273 -190.06222914032;-0.0002 -1.66560028750645 -167.733778074823 -192.64378947474;-0.00015 -1.63782115131122 -164.633970136487 -195.177817836697;-0.0001 -1.60963790725414 -161.493541229491 -197.663688992611;-5e-05 -1.58105750912897 -158.313266207676 -200.100789590972]  x5=0.000565541566995742  V1=[618 1.897e+04 1.855e+04;314.2 314.2 314.2;-0.004469 -0.02884 -1.594]  V2=[358.2 1.482e+04 1.449e+04;314.2 314.2 314.2;-0.2312 -0.2989 -1.864]  I1=[1.655 166 162.3;314.2 314.2 314.2;1.747 1.988 0.423]  I2=[2.42 258 252.2;314.2 314.2 314.2;-0.874 -0.7533 -2.318]  nHarmo=1  Measurements=None  Decoupling=off  VsMag0=0  VrMag0=0  VsAngle0=0  VrAngle0=0  IsMag0=0  IrMag0=0  IsAngle0=0  IrAngle0=0
      settings: LibrarySourceBlock=sps_lib/Power Grid Elements/Distributed Parameters Line
  Distributed Parameters Line6 : spsDistributedParametersLineLib/Distributed Parameters Line  Phases=3  Length=100  Frequency=60  Resistance=[0.01273 0.3864]  Inductance="[0.9337e-3  4.1264e-3]"  Capacitance=[12.74e-9 7.751e-9]  x1=[-0.0006 -53.5556902258853 1705.94068504693 4339.77814075333;-0.00055 -53.0136471064385 1773.23461186015 4310.87240894793;-0.0005 -52.4585236628284 1840.09101956638 4280.90303388059;-0.00045 -51.8904568634583 1906.49341234741 4249.87741004617;-0.0004 -51.3095868703106 1972.42540640641 4217.8031925531;-0.00035 -50.7160570043646 2037.87073401041 4184.68829523461;-0.0003 -50.1100137102333 2102.81324750411 4150.54088869611;-0.00025 -49.4916065200313 2167.23692329406 4115.3693982992;-0.0002 -48.8609880164793 2231.12586580225 4079.18250208285;-0.00015 -48.2183137952569 2294.46431138811 4041.98912862223;-0.0001 -47.5637424266116 2357.23663223794 4003.79845482571;-5e-05 -46.8974354162341 2419.42734022085 3964.61990367057]  x2=[-0.0006 -28.7204884369456 2975.17019854816 3835.35945269249;-0.00055 -26.8975754314509 3034.84212468875 3786.37675769128;-0.0005 -25.0680258516956 3093.76524894639 3736.45983088189;-0.00045 -23.2322911116623 3151.92503292185 3685.62098851908;-0.0004 -21.3908241514294 3209.3071265587 3633.87277432648;-0.00035 -19.5440793254149 3265.89737168397 3581.22795640162;-0.0003 -17.6925122902713 3321.68180550145 3527.69952406559;-0.00025 -15.8365798924587 3376.64666403682 3473.30068465809;-0.0002 -13.9767400555255 3430.77838553368 3418.04486027876;-0.00015 -12.1134516671221 3484.06361379975 3361.94568447547;-0.0001 -10.2471744657773 3536.48920150227 3305.0169988804;-5e-05 -8.37836892746478 3588.04221341195 3247.27284979489]  x3=[-0.0006 -0.590885266624386 23.4556585470751 59.2033447218124;-0.00055 -0.584862643241763 24.3737086362134 58.8060866725512;-0.0005 -0.578695713753408 25.2857448774574 58.3943191013379;-0.00045 -0.572385999756894 26.1915422395116 57.9681436056593;-0.0004 -0.565935058079736 27.0908772304306 57.5276653379419;-0.00035 -0.559344480395265 27.9835279527626 57.0729929796073;-0.0003 -0.552615892829907 28.8692741582986 56.6042387142566;-0.00025 -0.545750955561962 29.7478973024164 56.1215181999905;-0.0002 -0.53875136241198 30.6191805980021 55.6249505408729;-0.00015 -0.531618840424832 31.48290906894 55.1146582575433;-0.0001 -0.524355149443592 32.3388696031539 54.590767256987;-5e-05 -0.516962081675322 33.1868510051901 54.0534068014692]  x4=[-0.0006 0.464692630767085 -7.8479294598573 -28.1337372786828;-0.00055 0.461633565739402 -8.2837428669275 -27.9976335685444;-0.0005 0.458460599536944 -8.71751238439759 -27.8546218612605;-0.00045 0.455174515041644 -9.14913098612977 -27.70473744283;-0.0004 0.451776123045679 -9.57849217669251 -27.5480172949904;-0.00035 0.448266262051424 -10.0054900176367 -27.3845000860931;-0.0003 0.44464579806456 -10.4300191536344 -27.2142261615626;-0.00025 0.440915624380402 -10.8519748384737 -27.0372375339419;-0.0002 0.43707666136349 -11.2712529609031 -26.8535778725266;-0.00015 0.433129856220504 -11.6877500703199 -26.66329249259;-0.0001 0.429076182766558 -12.1013634022943 -26.4664283442022;-5e-05 0.424916641184919 -12.5119909039258 -26.2630340006462]  x5=0.000565541566995742  V1=[63.48 4624 4701;314.2 314.2 314.2;-0.9931 0.458 2.045]  V2=[119.3 4844 4924;314.2 314.2 314.2;-0.2322 0.7415 2.329]  I1=[0.7019 63.15 64.2;314.2 314.2 314.2;-0.9899 0.4607 2.048]  I2=[0.5025 28.89 29.37;314.2 314.2 314.2;1.972 -2.786 -1.199]  nHarmo=1  Measurements=None  Decoupling=off  VsMag0=0  VrMag0=0  VsAngle0=0  VrAngle0=0  IsMag0=0  IrMag0=0  IsAngle0=0  IrAngle0=0
      settings: LibrarySourceBlock=sps_lib/Power Grid Elements/Distributed Parameters Line
  Distributed Parameters Line7 : spsDistributedParametersLineLib/Distributed Parameters Line  Phases=3  Length=100  Frequency=60  Resistance=[0.01273 0.3864]  Inductance="[0.9337e-3  4.1264e-3]"  Capacitance=[12.74e-9 7.751e-9]  x1=[-0.0006 -95.754041116279 -7950.01158904029 -9140.45194809051;-0.00055 -93.3058973660337 -7802.93392827206 -9260.55415698169;-0.0005 -90.8347317817795 -7653.93101031483 -9378.37146270328;-0.00045 -88.3411540866474 -7503.03959940903 -9493.87479559802;-0.0004 -85.8257795336214 -7350.29692575247 -9607.03565694686;-0.00035 -83.2892287537342 -7195.74067631434 -9717.8261260005;-0.0003 -80.7321276029355 -7039.40898553651 -9826.21886686851;-0.00025 -78.1551070076716 -6881.34042592443 -9932.18713526398;-0.0002 -75.5588028092135 -6721.57399852996 -10035.7047851023;-0.00015 -72.9438556067728 -6560.14912332842 -10136.7462749524;-0.0001 -70.3109105994435 -6397.10562949233 -10235.2866743386;-5e-05 -67.6606174270086 -6232.4837455641 -10331.3016698917]  x2=[-0.0006 -85.5357957149079 -9626.19468720964 -5813.97373656627;-0.00055 -85.1374787262085 -9532.51047123588 -5960.54234228896;-0.0005 -84.7181553385728 -9436.47425094136 -6105.6402733782;-0.00045 -84.2779290137723 -9338.10972182641 -6249.23172909064;-0.0004 -83.8169083710654 -9237.44115386674 -6391.2812803832;-0.00035 -83.3352071603973 -9134.49338552515 -6531.75387865461;-0.0003 -82.8329442343338 -9029.29181762304 -6670.61486439319;-0.00025 -82.3102435187364 -8921.86240707313 -6807.82997572854;-0.0002 -81.7672339821854 -8812.23166047496 -6943.36535688512;-0.00015 -81.2040496041587 -8700.42662757483 -7077.1875665357;-0.0001 -80.6208293419744 -8586.47489459162 -7209.26358605247;-5e-05 -80.0177170965054 -8470.40457741035 -7339.5608276539]  x3=[-0.0006 0.781578660276759 82.4805734573994 29.2199547218989;-0.00055 0.781418698025991 82.0087456796244 30.480290263971;-0.0005 0.781065932404104 81.5166834709761 31.7331052505068;-0.00045 0.780520450450737 81.0045082404417 32.9780905681547;-0.0004 0.779782386755399 80.4723463595955 34.2149390354167;-0.00035 0.778851923424264 79.9203291314186 35.4433454784408;-0.0003 0.777729290035235 79.3485927579021 36.6630068063183;-0.00025 0.776414763581304 78.757278306441 37.8736220858667;-0.0002 0.774908668402202 78.1465316750283 39.0748926158805;-0.00015 0.773211376104379 77.5165035562564 40.2665220008316;-0.0001 0.771323305469313 76.8673494001363 41.4482162239998;-5e-05 0.76924492235018 76.1992293757426 42.6196837200177]  x4=[-0.0006 -1.04173882958928 -150.211602422387 -80.8486223789593;-0.00055 -1.0381655500713 -148.908363866387 -83.1378972138787;-0.0005 -1.03433611873825 -147.568384399766 -85.4066590166797;-0.00045 -1.03025148044501 -146.191994642407 -87.6543480043355;-0.0004 -1.02591264301494 -144.779534197888 -89.8804095932215;-0.00035 -1.02132067699128 -143.331351569689 -92.0842945359498;-0.0003 -1.01647671537291 -141.847804075202 -94.2654590568882;-0.00025 -1.0113819533349 -140.329257757575 -96.4233649863286;-0.0002 -1.00603764793353 -138.776087295387 -98.5574798932725;-0.00015 -1.0004451177962 -137.188675910211 -100.6672772168;-0.0001 -0.994605742796036 -135.567415272052 -102.752236395991;-5e-05 -0.988520963711441 -133.912705402713 -104.811842998366]  x5=0.000565541566995742  V1=[182.3 1.224e+04 1.196e+04;314.2 314.2 314.2;-0.5422 -0.6271 -2.192]  V2=[89.03 1.128e+04 1.103e+04;314.2 314.2 314.2;-1.279 -0.9416 -2.506]  I1=[0.7816 87.56 85.61;314.2 314.2 314.2;1.587 1.993 0.4285]  I2=[1.065 171 167.2;314.2 314.2 314.2;-1.352 -0.992 -2.557]  nHarmo=1  Measurements=None  Decoupling=off  VsMag0=0  VrMag0=0  VsAngle0=0  VrAngle0=0  IsMag0=0  IrMag0=0  IsAngle0=0  IrAngle0=0
      settings: LibrarySourceBlock=sps_lib/Power Grid Elements/Distributed Parameters Line
  Distributed Parameters Line8 : spsDistributedParametersLineLib/Distributed Parameters Line  Phases=3  Length=100  Frequency=60  Resistance=[0.01273 0.3864]  Inductance="[0.9337e-3  4.1264e-3]"  Capacitance=[12.74e-9 7.751e-9]  x1=[-0.0006 -3.34996941125908 -697.369780346788 -6144.14158944557;-0.00055 -0.116037454530759 -598.639966371315 -6153.51355579589;-0.0005 3.11792313270317 -499.762446941781 -6161.36723475331;-0.00045 6.35111441905858 -400.761618606571 -6167.70068854007;-0.0004 9.58273866296486 -301.661908338694 -6172.51235447122;-0.00035 12.8119985094957 -202.487767508799 -6175.80104534019;-0.0003 16.0380971871043 -103.26366585216 -6177.56594971172;-0.00025 19.2602387042152 -4.01408543114011 -6177.80663212206;-0.0002 22.477628045623 95.2364854053961 -6176.52303318643;-0.00015 25.6894713686504 194.463558064213 -6173.71546961365;-0.0001 28.8949761990175 293.642649749898 -6169.38463412804;-5e-05 32.0933516263723 392.749289505626 -6163.53159529844]  x2=[-0.0006 -52.8189100404899 -2873.25610929142 -4231.34825559502;-0.00055 -51.8687684469325 -2805.19349763607 -4274.55299250086;-0.0005 -50.9058290108899 -2736.43874646019 -4316.70304741732;-0.00045 -49.9303293232591 -2667.00881996984 -4357.78802044903;-0.0004 -48.9425100739914 -2596.92084896046 -4397.79777449369;-0.00035 -47.9426149927054 -2526.19212659017 -4436.72243774314;-0.0003 -46.9308907885507 -2454.84010411286 -4474.55240611919;-0.00025 -45.9075870893359 -2382.88238657243 -4511.27834564319;-0.0002 -44.8729563799368 -2310.33672845894 -4546.89119473911;-0.00015 -43.8272539399995 -2237.22102932802 -4581.38216646933;-0.0001 -42.7707377809536 -2163.55332938436 -4614.74275070265;-5e-05 -41.7036685823527 -2089.35180503063 -4646.96471621413]  x3=[-0.0006 0.881289797053524 59.9645909875103 53.0831369909919;-0.00055 0.875337778826808 59.1100382951137 53.9924862210409;-0.0005 0.869169784101126 58.2409010852503 54.8885136130219;-0.00045 0.862787334736885 57.3573938045215 55.7709980855832;-0.0004 0.856192005507961 56.4597344451284 56.6397218988864;-0.00035 0.849385423713154 55.5481444910862 57.4944707083293;-0.0003 0.842369268774673 54.6228488635755 58.3350336174331;-0.00025 0.835145271823763 53.684075865447 59.1612032298778;-0.0002 0.827715215273578 52.7320571248908 59.9727757006735;-0.00015 0.820080932379393 51.7670275382857 60.769550786457;-0.0001 0.812244306786278 50.7892252122422 61.5513318948982;-5e-05 0.804207272064335 49.798891404853 62.3179261332068]  x4=[-0.0006 -0.986887922118022 -75.2240362168441 -90.5885438251751;-0.00055 -0.975525845961934 -73.7664927081496 -91.724073551889;-0.0005 -0.963923073400461 -72.290748421171 -92.8369717359508;-0.00045 -0.952082467244118 -70.7971674737293 -93.9269637863862;-0.0004 -0.940006948985298 -69.2861183845742 -94.9937807639666;-0.00035 -0.927699498077442 -67.7579739824581 -96.0371594475659;-0.0003 -0.9151631511999 -66.2131113141461 -97.0568423991065;-0.00025 -0.902401001508681 -64.6519115513855 -98.0525780270777;-0.0002 -0.889416197873255 -63.0747598968569 -99.024120648613;-0.00015 -0.876211944099624 -61.4820454891316 -99.971230550108;-0.0001 -0.862791498139827 -59.8741613066575 -100.893674046366;-5e-05 -0.84915817128809 -58.2515040707972 -101.791223538258]  x5=0.000565541566995742  V1=[205.9 6319 6178;314.2 314.2 314.2;-0.005446 -0.03045 -1.595]  V2=[79.99 5180 5065;314.2 314.2 314.2;-0.7104 -0.5078 -2.073]  I1=[0.9566 80.65 78.85;314.2 314.2 314.2;1.981 2.383 0.8187]  I2=[1.219 119 116.3;314.2 314.2 314.2;-0.9326 -0.6042 -2.169]  nHarmo=1  Measurements=None  Decoupling=off  VsMag0=0  VrMag0=0  VsAngle0=0  VrAngle0=0  IsMag0=0  IrMag0=0  IsAngle0=0  IrAngle0=0
      settings: LibrarySourceBlock=sps_lib/Power Grid Elements/Distributed Parameters Line
  Distributed Parameters Line9 : spsDistributedParametersLineLib/Distributed Parameters Line  Phases=3  Length=100  Frequency=60  Resistance=[0.01273 0.3864]  Inductance="[0.9337e-3  4.1264e-3]"  Capacitance=[12.74e-9 7.751e-9]  x1=[-0.0006 -52.8189100404899 -2873.25610929142 -4231.34825559502;-0.00055 -51.8687684469325 -2805.19349763607 -4274.55299250086;-0.0005 -50.9058290108899 -2736.43874646019 -4316.70304741732;-0.00045 -49.9303293232591 -2667.00881996984 -4357.78802044903;-0.0004 -48.9425100739914 -2596.92084896046 -4397.79777449369;-0.00035 -47.9426149927054 -2526.19212659017 -4436.72243774314;-0.0003 -46.9308907885507 -2454.84010411286 -4474.55240611919;-0.00025 -45.9075870893359 -2382.88238657243 -4511.27834564319;-0.0002 -44.8729563799368 -2310.33672845894 -4546.89119473911;-0.00015 -43.8272539399995 -2237.22102932802 -4581.38216646933;-0.0001 -42.7707377809536 -2163.55332938436 -4614.74275070265;-5e-05 -41.7036685823527 -2089.35180503063 -4646.96471621413]  x2=[-0.0006 -42.3870045605464 -3784.43185018062 -3134.5391909349;-0.00055 -42.3225832883335 -3733.96377837267 -3191.97617660435;-0.0005 -42.2477195519808 -3682.57440687489 -3248.62558991479;-0.00045 -42.1624318229947 -3630.27641524577 -3304.47345347115;-0.0004 -42.0667411448463 -3577.08270723217 -3359.50598764876;-0.00035 -41.9606711277786 -3523.00640758561 -3413.70961399328;-0.0003 -41.8442479429811 -3468.06085882384 -3467.07095857099;-0.00025 -41.7175003161327 -3412.25961793888 -3519.57685526856;-0.0002 -41.5804595203135 -3355.61645305192 -3571.21434904166;-0.00015 -41.4331593682895 -3298.14534001634 -3621.97069911135;-0.0001 -41.2756362041691 -3239.86045896931 -3671.83338210776;-5e-05 -41.1079288944358 -3180.77619083311 -3720.79009515995]  x3=[-0.0006 0.335498596394081 25.5648916047918 17.1231340702837;-0.00055 0.335922092646544 25.2890565106852 17.5120191558684;-0.0005 0.336262705149156 25.0069817202929 17.8965834127642;-0.00045 0.336520349860881 24.7187368313486 18.2767319554953;-0.0004 0.336694963211739 24.4243929639656 18.652370988097;-0.00035 0.336786502118499 24.1240227430887 19.0234078272588;-0.0003 0.336794943995306 23.8177002805755 19.3897509251925;-0.00025 0.336720286759254 23.50550115691 19.7513098922206;-0.0002 0.336562548830897 23.1875024025543 20.1079955190779;-0.00015 0.33632176912971 22.8637824789429 20.4597197989233;-0.0001 0.33599800706448 22.5344212591229 20.8063959490537;-5e-05 0.335591342518654 22.199500008047 21.1479384323165]  x4=[-0.0006 -0.468488862237583 -51.5684690160704 -42.9438340064732;-0.00055 -0.467752874465577 -50.8770541001197 -43.7264473760195;-0.0005 -0.466901475670933 -50.1730860323596 -44.4982718989687;-0.00045 -0.465934875923563 -49.456738506377 -45.2591171391687;-0.0004 -0.464853313717493 -48.7281882702051 -46.0087953694413;-0.00035 -0.463657055912013 -47.9876150827129 -46.7471216179009;-0.0003 -0.462346397665836 -47.2352016692533 -47.4739137135935;-0.00025 -0.460921662364272 -46.4711336765772 -48.1889923314447;-0.0002 -0.459383201539439 -45.6955996270289 -48.8921810365054;-0.00015 -0.457731394783524 -44.9087908720306 -49.5833063274848;-0.0001 -0.455966649655128 -44.1109015448693 -50.2621976795588;-5e-05 -0.454089401578706 -43.3021285127973 -50.9286875864449]  x5=0.000565541566995742  V1=[79.99 5180 5065;314.2 314.2 314.2;-0.7104 -0.5078 -2.073]  V2=[42.55 4945 4835;314.2 314.2 314.2;-1.471 -0.7913 -2.356]  I1=[0.3368 30.9 30.21;314.2 314.2 314.2;1.494 2.247 0.6827]  I2=[0.4705 67.54 66.03;314.2 314.2 314.2;-1.468 -0.7886 -2.353]  nHarmo=1  Measurements=None  Decoupling=off  VsMag0=0  VrMag0=0  VsAngle0=0  VrAngle0=0  IsMag0=0  IrMag0=0  IsAngle0=0  IrAngle0=0
      settings: LibrarySourceBlock=sps_lib/Power Grid Elements/Distributed Parameters Line
  Load Flow Bus : spsLoadFlowBusLib/Load Flow Bus  LConnTagsString=a|b|c  RConnTagsString=a|b|c  Phases=ABC  Connectors=on both sides  ID=BUS_2  Vbase=11e3  Vref=1  Vangle=0  VLF=1  VLFb=1  VLFc=1  angleLF=0  angleLFb=0  angleLFc=0
  Load Flow Bus1 : spsLoadFlowBusLib/Load Flow Bus  LConnTagsString=a|b|c  RConnTagsString=a|b|c  Phases=ABC  Connectors=on both sides  ID=BUS_1  Vbase=11e3  Vref=1  Vangle=0  VLF=1  VLFb=1  VLFc=1  angleLF=0  angleLFb=0  angleLFc=0
  Load Flow Bus10 : spsLoadFlowBusLib/Load Flow Bus  LConnTagsString=a|b|c  RConnTagsString=a|b|c  Phases=ABC  Connectors=on both sides  ID=BUS_11  Vbase=11e3  Vref=1  Vangle=0  VLF=1  VLFb=1  VLFc=1  angleLF=0  angleLFb=0  angleLFc=0
  Load Flow Bus11 : spsLoadFlowBusLib/Load Flow Bus  LConnTagsString=a|b|c  RConnTagsString=a|b|c  Phases=ABC  Connectors=on both sides  ID=BUS_12  Vbase=11e3  Vref=1  Vangle=0  VLF=1  VLFb=1  VLFc=1  angleLF=0  angleLFb=0  angleLFc=0
  Load Flow Bus12 : spsLoadFlowBusLib/Load Flow Bus  LConnTagsString=a|b|c  RConnTagsString=a|b|c  Phases=ABC  Connectors=on both sides  ID=BUS_13  Vbase=11e3  Vref=1  Vangle=0  VLF=1  VLFb=1  VLFc=1  angleLF=0  angleLFb=0  angleLFc=0
  Load Flow Bus2 : spsLoadFlowBusLib/Load Flow Bus  LConnTagsString=a|b|c  RConnTagsString=a|b|c  Phases=ABC  Connectors=on both sides  ID=BUS_3  Vbase=11e3  Vref=1  Vangle=0  VLF=1  VLFb=1  VLFc=1  angleLF=0  angleLFb=0  angleLFc=0
  Load Flow Bus3 : spsLoadFlowBusLib/Load Flow Bus  LConnTagsString=a|b|c  RConnTagsString=a|b|c  Phases=ABC  Connectors=on both sides  ID=BUS_4  Vbase=11e3  Vref=1  Vangle=0  VLF=1  VLFb=1  VLFc=1  angleLF=0  angleLFb=0  angleLFc=0
  Load Flow Bus4 : spsLoadFlowBusLib/Load Flow Bus  LConnTagsString=a|b|c  RConnTagsString=a|b|c  Phases=ABC  Connectors=on both sides  ID=BUS_5  Vbase=11e3  Vref=1  Vangle=0  VLF=1  VLFb=1  VLFc=1  angleLF=0  angleLFb=0  angleLFc=0
  Load Flow Bus5 : spsLoadFlowBusLib/Load Flow Bus  LConnTagsString=a|b|c  RConnTagsString=a|b|c  Phases=ABC  Connectors=on both sides  ID=BUS_8  Vbase=11e3  Vref=1  Vangle=0  VLF=1  VLFb=1  VLFc=1  angleLF=0  angleLFb=0  angleLFc=0
  Load Flow Bus6 : spsLoadFlowBusLib/Load Flow Bus  LConnTagsString=a|b|c  RConnTagsString=a|b|c  Phases=ABC  Connectors=on both sides  ID=BUS_6  Vbase=11e3  Vref=1  Vangle=0  VLF=1  VLFb=1  VLFc=1  angleLF=0  angleLFb=0  angleLFc=0
  Load Flow Bus7 : spsLoadFlowBusLib/Load Flow Bus  LConnTagsString=a|b|c  RConnTagsString=a|b|c  Phases=ABC  Connectors=on both sides  ID=BUS_7  Vbase=11e3  Vref=1  Vangle=0  VLF=1  VLFb=1  VLFc=1  angleLF=0  angleLFb=0  angleLFc=0
  Load Flow Bus8 : spsLoadFlowBusLib/Load Flow Bus  LConnTagsString=a|b|c  RConnTagsString=a|b|c  Phases=ABC  Connectors=on both sides  ID=BUS_9  Vbase=11e3  Vref=1  Vangle=0  VLF=1  VLFb=1  VLFc=1  angleLF=0  angleLFb=0  angleLFc=0
  Load Flow Bus9 : spsLoadFlowBusLib/Load Flow Bus  LConnTagsString=a|b|c  RConnTagsString=a|b|c  Phases=ABC  Connectors=on both sides  ID=BUS_10  Vbase=11e3  Vref=1  Vangle=0  VLF=1  VLFb=1  VLFc=1  angleLF=0  angleLFb=0  angleLFc=0
  "Power (3ph, Phasor)" : spsPower3phPhasorLib/Power (3ph, Phasor)
      settings: LibrarySourceBlock=|
      | sps_lib/Sensors and Measurements/Power
      | (3ph, Phasor)
  Scope : Scope
  Scope1 : Scope
  Three-Phase Series RLC Load{1..9,11..12,14..15} (13 alike) : spsThreePhaseSeriesRLCLoadLib/Three-Phase Series RLC Load  LConnTagsString=A|B|C  Configuration=Y (grounded)  NominalVoltage=1000  Vabc=[1e3 1e3 1e3]  Vabcp=[1e3 1e3 1e3]  NominalFrequency=60  UnbalancedPower=off  ActivePower=10e3  InductivePower=100  CapacitivePower=100  Pabc=[10e3 9e3 11e3]  QLabc=[100 90 110]  QCabc=[100 90 110]  Pabcp=[10e3 9e3 11e3]  QLabcp=[100 90 110]  QCabcp=[100 90 110]  Measurements=None  LoadType=constant Z
  Three-Phase Series RLC Load13 : spsThreePhaseSeriesRLCLoadLib/Three-Phase Series RLC Load  LConnTagsString=A|B|C  Configuration=Y (grounded)  NominalVoltage=11000  Vabc=[1e3 1e3 1e3]  Vabcp=[1e3 1e3 1e3]  NominalFrequency=50  UnbalancedPower=off  ActivePower=10e3  InductivePower=10000  CapacitivePower=0  Pabc=[10e3 9e3 11e3]  QLabc=[100 90 110]  QCabc=[100 90 110]  Pabcp=[10e3 9e3 11e3]  QLabcp=[100 90 110]  QCabcp=[100 90 110]  Measurements=None  LoadType=constant PQ
  Three-Phase Transformer (Two Windings) : spsThreePhaseTransformerTwoWindingsLib/Three-Phase Transformer (Two Windings)  Winding1Connection=Yg  Winding2Connection=Yg  CoreType=Three single-phase transformers  SetSaturation=off  Hysteresis=off  DataFile='hysteresis'  SetInitialFlux=off  Measurements=None  UNITS=pu  NominalPower=[ 250e6 , 60 ]  Winding1=[ 66e3 , 0.002 , 0.08 ]  Winding2=[ 33e3 , 0.002 , 0.08 ]  Rm=500  Lm=500  L0=0.5  Saturation=[ 0,0 ; 0.0024,1.2 ; 1.0,1.52 ]  InitialFluxes=[ 0.8 , -0.8 , 0.7 ]  BreakLoop=off  DiscreteSolver=Trapezoidal iterative  DataType=off  TransfoNumber=1
  Three-Phase Transformer (Two Windings){1..5} (5 alike) : spsThreePhaseTransformerTwoWindingsLib/Three-Phase Transformer (Two Windings)  Winding1Connection=Yg  Winding2Connection=Yg  CoreType=Three single-phase transformers  SetSaturation=off  Hysteresis=off  DataFile='hysteresis'  SetInitialFlux=off  Measurements=None  UNITS=pu  NominalPower=[ 250e6 , 60 ]  Winding1=[ 33e3 , 0.002 , 0.08 ]  Winding2=[ 11e3 , 0.002 , 0.08 ]  Rm=500  Lm=500  L0=0.5  Saturation=[ 0,0 ; 0.0024,1.2 ; 1.0,1.52 ]  InitialFluxes=[ 0.8 , -0.8 , 0.7 ]  BreakLoop=off  DiscreteSolver=Trapezoidal iterative  DataType=off  TransfoNumber=1
  Three-Phase V-I Measurement{,1..18,21} (20 alike) : spsThreePhaseVIMeasurementLib/Three-Phase V-I Measurement  VoltageMeasurement=phase-to-ground  SetLabelV=off  LabelV=Vabc  Vpu=off  VpuLL=off  CurrentMeasurement=yes  SetLabelI=off  LabelI=Iabc  Ipu=off  Pbase=100e6  Vbase=500e3  OutputType=Complex  PhasorSimulation=off  PSBequivalent=0
  Three-Phase Source : spsThreePhaseSourceLib/Three-Phase Source  InternalConnection=Yg  VoltagePhases=off  Voltage=66e3  PhaseAngle=0  Voltage_phases=[25e3 25e3 25e3]/sqrt(3)  PhaseAngles_phases=[0 -120 +120]  Frequency=50  NonIdealSource=on  SpecifyImpedance=off  Resistance=0.8929  Inductance=16.58e-3  ShortCircuitLevel=100e6  BaseVoltage=66e3  XRratio=7  BusType=swing  Pref=10e3  Qref=0  Prefabc=[10e3, 10e3, 10e3]  Qrefabc=[0, 0, 0]  Qmin=-inf  Qmax=inf
  powergui : sps_lib/powergui  Priority=1  SimulationMode=Discrete  SampleTime=50e-6  frequency=60  Iterations=50  frequencyindice=60  Pbase=100e6  ErrMax=1e-4  UnitsV=kV  UnitsW=MW  buscounter=0  FunctionMessages=off  echomessages=off  EnableUseOfTLC=off  CurrentSourceSwitches=off  DisableSnubberDevices=off  DisableRonSwitches=off  DisableVfSwitches=off  DisplayEquations=off  AutomaticDiscreteSolvers=off  SolverType=Tustin/Backward Euler (TBE)  Interpol=off  ExternalGateDelay=off  methode=off  Ts=100  x0status=blocks  SPID=on  SwTol=0  HookPort=off  NonlinearTolerance=1e-4  nMaxIteration=100  ContinueOnMaxIteration=off  RestoreLinks=warning  ResistiveCurrentMeasurement=off  Frange=[0:2:500]  Ylog=off  Xlog=on  ShowGrid=off  save=off  variable=ZData  structure=0  ZoomFFT=off  StartTime=0.0  cycles=1  DisplayStyle=1  fundamental=60  FreqAxis=off  MaxFrequency=1000  frequencyindicesteady=1  RmsSteady=1  display=off
  wires:
  Three-Phase V-I Measurement9/1 -> Scope1/1
  Three-Phase V-I Measurement9/2 -> Scope/1
  "Power (3ph, Phasor)"/1 -> Display/1
  "Power (3ph, Phasor)"/2 -> Display1/1
  Three-Phase V-I Measurement8/1 -> "Power (3ph, Phasor)"/1
  Three-Phase V-I Measurement8/2 -> "Power (3ph, Phasor)"/2
  connections:
  Three-Phase V-I Measurement/LConn3 -- Three-Phase Source/RConn3
  Three-Phase Source/RConn2 -- Three-Phase V-I Measurement/LConn2
  Three-Phase Source/RConn1 -- Three-Phase V-I Measurement/LConn1
  Three-Phase V-I Measurement1/LConn3 -- Distributed Parameters Line/RConn3 -- Three-Phase Transformer (Two Windings)1/LConn3
  Distributed Parameters Line/RConn2 -- Three-Phase Transformer (Two Windings)1/LConn2 -- Three-Phase V-I Measurement1/LConn2
  Distributed Parameters Line/RConn1 -- Three-Phase V-I Measurement1/LConn1 -- Three-Phase Transformer (Two Windings)1/LConn1
  Three-Phase V-I Measurement/RConn1 -- Three-Phase Transformer (Two Windings)/LConn1
  Three-Phase V-I Measurement/RConn2 -- Three-Phase Transformer (Two Windings)/LConn2
  Three-Phase V-I Measurement/RConn3 -- Three-Phase Transformer (Two Windings)/LConn3
  Three-Phase V-I Measurement2/RConn2 -- Distributed Parameters Line/LConn2
  Distributed Parameters Line/LConn3 -- Three-Phase V-I Measurement2/RConn3
  Three-Phase V-I Measurement3/LConn3 -- Three-Phase Transformer (Two Windings)2/LConn3 -- Distributed Parameters Line1/RConn3
  Distributed Parameters Line1/RConn2 -- Three-Phase Transformer (Two Windings)2/LConn2 -- Three-Phase V-I Measurement3/LConn2
  Distributed Parameters Line1/RConn1 -- Three-Phase Transformer (Two Windings)2/LConn1 -- Three-Phase V-I Measurement3/LConn1
  Three-Phase V-I Measurement6/LConn3 -- Three-Phase Transformer (Two Windings)4/LConn3 -- Distributed Parameters Line4/RConn3
  Distributed Parameters Line4/RConn2 -- Three-Phase Transformer (Two Windings)4/LConn2 -- Three-Phase V-I Measurement6/LConn2
  Distributed Parameters Line4/RConn1 -- Three-Phase Transformer (Two Windings)4/LConn1 -- Three-Phase V-I Measurement6/LConn1
  Three-Phase V-I Measurement7/LConn3 -- Three-Phase Transformer (Two Windings)3/LConn3 -- Distributed Parameters Line5/RConn3
  Distributed Parameters Line5/RConn2 -- Three-Phase Transformer (Two Windings)3/LConn2 -- Three-Phase V-I Measurement7/LConn2
  Distributed Parameters Line5/RConn1 -- Three-Phase Transformer (Two Windings)3/LConn1 -- Three-Phase V-I Measurement7/LConn1
  Three-Phase V-I Measurement9/LConn3 -- Distributed Parameters Line7/RConn3 -- Three-Phase Transformer (Two Windings)5/LConn3
  Distributed Parameters Line7/RConn2 -- Three-Phase Transformer (Two Windings)5/LConn2 -- Three-Phase V-I Measurement9/LConn2
  Distributed Parameters Line7/RConn1 -- Three-Phase Transformer (Two Windings)5/LConn1 -- Three-Phase V-I Measurement9/LConn1
  Distributed Parameters Line1/LConn1 -- Three-Phase V-I Measurement1/RConn1
  Distributed Parameters Line1/LConn2 -- Three-Phase V-I Measurement1/RConn2
  Distributed Parameters Line1/LConn3 -- Three-Phase V-I Measurement1/RConn3
  Distributed Parameters Line5/LConn2 -- Three-Phase V-I Measurement3/RConn2
  Distributed Parameters Line5/LConn1 -- Three-Phase V-I Measurement3/RConn1
  Distributed Parameters Line5/LConn3 -- Three-Phase V-I Measurement3/RConn3
  Three-Phase V-I Measurement2/RConn1 -- Distributed Parameters Line/LConn1
  Distributed Parameters Line4/LConn1 -- Three-Phase V-I Measurement7/RConn1
  Distributed Parameters Line4/LConn2 -- Three-Phase V-I Measurement7/RConn2
  Distributed Parameters Line4/LConn3 -- Three-Phase V-I Measurement7/RConn3
  Distributed Parameters Line7/LConn1 -- Three-Phase V-I Measurement6/RConn1
  Distributed Parameters Line7/LConn2 -- Three-Phase V-I Measurement6/RConn2
  Distributed Parameters Line7/LConn3 -- Three-Phase V-I Measurement6/RConn3
  Three-Phase Series RLC Load3/LConn2 -- Three-Phase V-I Measurement9/RConn2
  Three-Phase Series RLC Load3/LConn1 -- Three-Phase V-I Measurement9/RConn1
  Three-Phase Series RLC Load3/LConn3 -- Three-Phase V-I Measurement9/RConn3
  Distributed Parameters Line2/LConn2 -- Load Flow Bus/RConn2 -- Three-Phase Transformer (Two Windings)1/RConn2
  Distributed Parameters Line2/LConn3 -- Load Flow Bus/RConn3 -- Three-Phase Transformer (Two Windings)1/RConn3
  Distributed Parameters Line2/LConn1 -- Load Flow Bus/RConn1 -- Three-Phase Transformer (Two Windings)1/RConn1
  Three-Phase Transformer (Two Windings)/RConn3 -- Three-Phase V-I Measurement2/LConn3
  Three-Phase Transformer (Two Windings)/RConn1 -- Three-Phase V-I Measurement2/LConn1
  Three-Phase V-I Measurement2/LConn2 -- Three-Phase Transformer (Two Windings)/RConn2
  Load Flow Bus1/RConn2 -- Distributed Parameters Line19/LConn2
  Load Flow Bus1/RConn1 -- Distributed Parameters Line19/LConn1
  Load Flow Bus1/RConn3 -- Distributed Parameters Line19/LConn3
  Three-Phase Series RLC Load8/LConn2 -- Three-Phase V-I Measurement21/RConn2 -- Distributed Parameters Line19/RConn2
  Three-Phase V-I Measurement21/RConn3 -- Distributed Parameters Line19/RConn1 -- Three-Phase Series RLC Load8/LConn3
  Three-Phase V-I Measurement5/LConn2 -- Load Flow Bus2/RConn2
  Three-Phase V-I Measurement5/LConn1 -- Load Flow Bus2/RConn1
  Three-Phase V-I Measurement5/LConn3 -- Load Flow Bus2/RConn3
  Distributed Parameters Line3/LConn2 -- Three-Phase Series RLC Load12/LConn2 -- Three-Phase Series RLC Load12/LConn1 -- Three-Phase V-I Measurement5/RConn2
  Three-Phase V-I Measurement5/RConn1 -- Distributed Parameters Line3/LConn1
  Three-Phase V-I Measurement5/RConn3 -- Three-Phase Series RLC Load12/LConn3 -- Distributed Parameters Line3/LConn3
  Load Flow Bus2/LConn1 -- Distributed Parameters Line2/RConn1
  Load Flow Bus2/LConn2 -- Distributed Parameters Line2/RConn2
  Load Flow Bus2/LConn3 -- Distributed Parameters Line2/RConn3
  Load Flow Bus3/RConn2 -- Three-Phase V-I Measurement8/LConn2
  Load Flow Bus3/RConn1 -- Three-Phase V-I Measurement8/LConn1
  Load Flow Bus3/RConn3 -- Three-Phase V-I Measurement8/LConn3
  Load Flow Bus3/LConn2 -- Distributed Parameters Line3/RConn2
  Distributed Parameters Line3/RConn1 -- Load Flow Bus3/LConn1
  Distributed Parameters Line3/RConn3 -- Load Flow Bus3/LConn3
  Load Flow Bus6/LConn1 -- Distributed Parameters Line8/RConn1
  Load Flow Bus6/LConn3 -- Distributed Parameters Line8/RConn3
  Three-Phase V-I Measurement12/RConn3 -- Three-Phase Series RLC Load15/LConn3 -- Distributed Parameters Line9/LConn3
  Three-Phase V-I Measurement12/RConn1 -- Distributed Parameters Line9/LConn1 -- Three-Phase Series RLC Load15/LConn1
  Load Flow Bus7/LConn2 -- Distributed Parameters Line9/RConn2
  Load Flow Bus7/RConn2 -- Three-Phase V-I Measurement13/LConn2
  Three-Phase V-I Measurement12/LConn1 -- Load Flow Bus6/RConn1
  Load Flow Bus6/LConn2 -- Distributed Parameters Line8/RConn2
  Three-Phase V-I Measurement12/LConn3 -- Load Flow Bus6/RConn3
  Distributed Parameters Line9/LConn2 -- Three-Phase Series RLC Load15/LConn2 -- Three-Phase V-I Measurement12/RConn2
  Three-Phase V-I Measurement12/LConn2 -- Load Flow Bus6/RConn2
  Distributed Parameters Line9/RConn1 -- Load Flow Bus7/LConn1
  Distributed Parameters Line9/RConn3 -- Load Flow Bus7/LConn3
  Three-Phase V-I Measurement10/LConn2 -- Load Flow Bus4/LConn2
  Three-Phase V-I Measurement10/LConn1 -- Load Flow Bus4/LConn1
  Three-Phase V-I Measurement10/LConn3 -- Load Flow Bus4/LConn3
  Three-Phase Transformer (Two Windings)2/RConn1 -- Distributed Parameters Line8/LConn1 -- Load Flow Bus4/RConn1
  Three-Phase Transformer (Two Windings)2/RConn2 -- Distributed Parameters Line8/LConn2 -- Load Flow Bus4/RConn2
  Three-Phase Transformer (Two Windings)2/RConn3 -- Distributed Parameters Line8/LConn3 -- Load Flow Bus4/RConn3
  Three-Phase V-I Measurement11/LConn2 -- Load Flow Bus5/LConn2
  Three-Phase V-I Measurement11/LConn1 -- Load Flow Bus5/LConn1
  Three-Phase V-I Measurement11/LConn3 -- Load Flow Bus5/LConn3
  Three-Phase V-I Measurement14/LConn2 -- Load Flow Bus8/LConn2
  Three-Phase V-I Measurement14/LConn1 -- Load Flow Bus8/LConn1
  Three-Phase V-I Measurement14/LConn3 -- Load Flow Bus8/LConn3
  Distributed Parameters Line6/LConn2 -- Load Flow Bus8/RConn2
  Load Flow Bus8/RConn3 -- Distributed Parameters Line6/LConn1
  Load Flow Bus8/RConn1 -- Distributed Parameters Line6/LConn3
  Load Flow Bus5/RConn2 -- Three-Phase Transformer (Two Windings)3/RConn2
  Load Flow Bus5/RConn3 -- Three-Phase Transformer (Two Windings)3/RConn3
  Load Flow Bus5/RConn1 -- Three-Phase Transformer (Two Windings)3/RConn1
  Distributed Parameters Line6/RConn3 -- Three-Phase V-I Measurement11/RConn1 -- Three-Phase Series RLC Load7/LConn1
  Distributed Parameters Line6/RConn2 -- Three-Phase V-I Measurement11/RConn2 -- Three-Phase Series RLC Load7/LConn2
  Distributed Parameters Line6/RConn1 -- Three-Phase Series RLC Load7/LConn3 -- Three-Phase V-I Measurement11/RConn3
  Three-Phase V-I Measurement15/LConn3 -- Load Flow Bus9/LConn3
  Three-Phase V-I Measurement15/LConn1 -- Load Flow Bus9/LConn1
  Three-Phase V-I Measurement15/LConn2 -- Load Flow Bus9/LConn2
  Three-Phase V-I Measurement16/LConn3 -- Load Flow Bus10/LConn3
  Three-Phase V-I Measurement16/LConn2 -- Load Flow Bus10/LConn2
  Distributed Parameters Line10/RConn2 -- Three-Phase Series RLC Load4/LConn2 -- Three-Phase V-I Measurement15/RConn2
  Load Flow Bus10/LConn1 -- Three-Phase V-I Measurement16/LConn1
  Distributed Parameters Line10/LConn1 -- Load Flow Bus10/RConn3
  Distributed Parameters Line10/LConn3 -- Load Flow Bus10/RConn1
  Distributed Parameters Line10/LConn2 -- Load Flow Bus10/RConn2
  Distributed Parameters Line10/RConn3 -- Three-Phase Series RLC Load4/LConn3 -- Three-Phase V-I Measurement15/RConn3
  Distributed Parameters Line10/RConn1 -- Three-Phase V-I Measurement15/RConn1 -- Three-Phase Series RLC Load4/LConn1
  Load Flow Bus9/RConn3 -- Three-Phase Transformer (Two Windings)4/RConn3 -- Distributed Parameters Line11/RConn1
  Load Flow Bus9/RConn1 -- Distributed Parameters Line11/RConn3 -- Three-Phase Transformer (Two Windings)4/RConn1
  Load Flow Bus9/RConn2 -- Distributed Parameters Line11/RConn2 -- Three-Phase Transformer (Two Windings)4/RConn2
  Load Flow Bus7/RConn1 -- Three-Phase V-I Measurement13/LConn1
  Load Flow Bus7/RConn3 -- Three-Phase V-I Measurement13/LConn3
  Distributed Parameters Line11/LConn1 -- Load Flow Bus11/RConn3
  Load Flow Bus11/LConn1 -- Three-Phase V-I Measurement17/LConn1
  Three-Phase V-I Measurement17/LConn3 -- Load Flow Bus11/LConn3
  Distributed Parameters Line11/LConn2 -- Load Flow Bus11/RConn2
  Distributed Parameters Line11/LConn3 -- Load Flow Bus11/RConn1
  Three-Phase V-I Measurement17/LConn2 -- Load Flow Bus11/LConn2
  Three-Phase V-I Measurement18/LConn2 -- Load Flow Bus12/LConn2
  Distributed Parameters Line12/LConn3 -- Load Flow Bus12/RConn1
  Load Flow Bus12/LConn1 -- Three-Phase V-I Measurement18/LConn1
  Distributed Parameters Line12/LConn1 -- Load Flow Bus12/RConn3
  Distributed Parameters Line12/LConn2 -- Load Flow Bus12/RConn2
  Three-Phase V-I Measurement18/LConn3 -- Load Flow Bus12/LConn3
  Distributed Parameters Line12/RConn2 -- Three-Phase Transformer (Two Windings)5/RConn2
  Distributed Parameters Line12/RConn1 -- Three-Phase Transformer (Two Windings)5/RConn3
  Distributed Parameters Line12/RConn3 -- Three-Phase Transformer (Two Windings)5/RConn1
  Three-Phase Series RLC Load5/LConn2 -- Three-Phase V-I Measurement18/RConn2
  Three-Phase Series RLC Load1/LConn2 -- Three-Phase V-I Measurement17/RConn2
  Three-Phase Series RLC Load2/LConn2 -- Three-Phase V-I Measurement16/RConn2
  Three-Phase V-I Measurement4/LConn2 -- Load Flow Bus1/LConn2
  Load Flow Bus1/LConn3 -- Three-Phase V-I Measurement4/LConn3
  Three-Phase V-I Measurement4/LConn1 -- Load Flow Bus1/LConn1
  Three-Phase Series RLC Load14/LConn2 -- Three-Phase V-I Measurement4/RConn2
  Three-Phase Series RLC Load14/LConn1 -- Three-Phase V-I Measurement4/RConn1
  Three-Phase Series RLC Load14/LConn3 -- Three-Phase V-I Measurement4/RConn3
  Load Flow Bus/LConn2 -- Three-Phase V-I Measurement21/LConn2
  Load Flow Bus/LConn1 -- Three-Phase V-I Measurement21/LConn1
  Three-Phase V-I Measurement21/LConn3 -- Load Flow Bus/LConn3
  Distributed Parameters Line19/RConn3 -- Three-Phase Series RLC Load8/LConn1 -- Three-Phase V-I Measurement21/RConn1
  Three-Phase Series RLC Load13/LConn2 -- Three-Phase V-I Measurement8/RConn2
  Three-Phase V-I Measurement8/RConn1 -- Three-Phase Series RLC Load13/LConn1
  Three-Phase V-I Measurement8/RConn3 -- Three-Phase Series RLC Load13/LConn3
  Three-Phase Series RLC Load9/LConn2 -- Three-Phase V-I Measurement10/RConn2
  Three-Phase V-I Measurement10/RConn1 -- Three-Phase Series RLC Load9/LConn1
  Three-Phase V-I Measurement10/RConn3 -- Three-Phase Series RLC Load9/LConn3
  Three-Phase Series RLC Load11/LConn2 -- Three-Phase V-I Measurement13/RConn2
  Three-Phase V-I Measurement13/RConn1 -- Three-Phase Series RLC Load11/LConn1
  Three-Phase V-I Measurement13/RConn3 -- Three-Phase Series RLC Load11/LConn3
  Three-Phase Series RLC Load6/LConn2 -- Three-Phase V-I Measurement14/RConn2
  Three-Phase V-I Measurement14/RConn1 -- Three-Phase Series RLC Load6/LConn1
  Three-Phase V-I Measurement14/RConn3 -- Three-Phase Series RLC Load6/LConn3
  Three-Phase V-I Measurement18/RConn3 -- Three-Phase Series RLC Load5/LConn3
  Three-Phase V-I Measurement18/RConn1 -- Three-Phase Series RLC Load5/LConn1
  Three-Phase Series RLC Load1/LConn1 -- Three-Phase V-I Measurement17/RConn1
  Three-Phase Series RLC Load1/LConn3 -- Three-Phase V-I Measurement17/RConn3
  Three-Phase Series RLC Load2/LConn3 -- Three-Phase V-I Measurement16/RConn3
  Three-Phase Series RLC Load2/LConn1 -- Three-Phase V-I Measurement16/RConn1
